simulink model "BaseEngineController_LS"  (Simulink 7.7)
settings: Solver=FixedStepDiscrete  StartTime=0.0  StopTime=10.0  RelTol=1e-3
PreLoadFcn:
  | try, eval([bdroot '_setup']); catch, eval('model_setup', ''); end
InitFcn:
  | try, eval([bdroot '_setup']); catch, eval('model_setup', ''); end
undefined symbols (not defined in the file): ECU555, High, motohawk_build_version, motohawk_trunc_name, motohawk_vardec_config_group, motohawk_vardec_path, True
libraries: MotoHawk_lib x1418, motohawk_control_primitives_lib x183, motohawk_engine_lib x32, simulink x21, motohawk_annotations_lib x9, AutoDoc_lib x8, simulink_extras x4, motohawk_ccp_examples_lib x1, motohawk_control_primitives_motoshare_lib x1
(part 14 of 27)

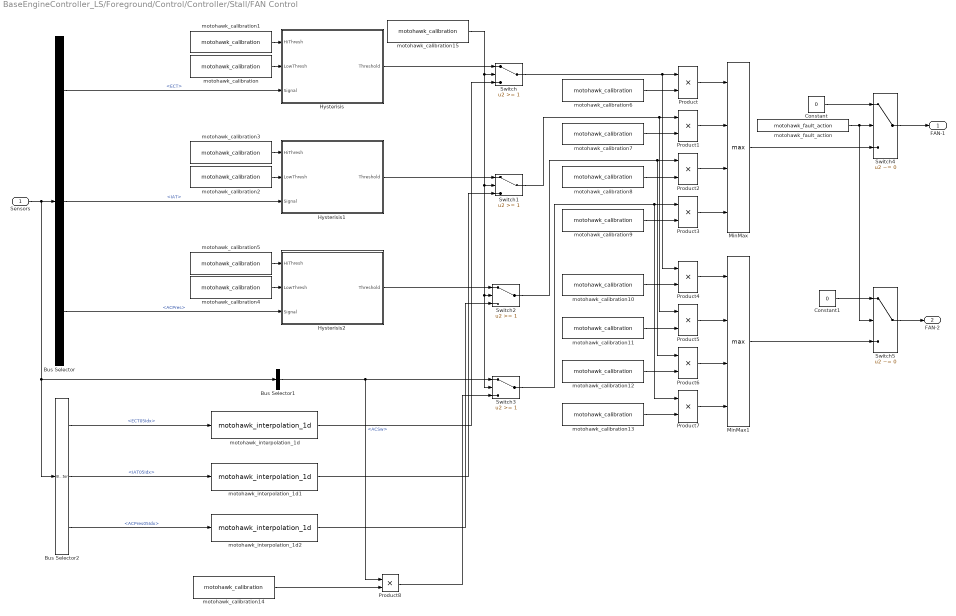
== system BaseEngineController_LS/Foreground/Control/Controller/Stall/FAN Control ==
  Sensors : Inport
  Bus Selector : BusSelector  OutputSignals=Raw.NonLinearSensors.ECT,Raw.NonLinearSensors.IAT,Raw.LinearSensors.ACPres
  Bus Selector1 : BusSelector  OutputSignals=Raw.Digital.ACSw
  Bus Selector2 : BusSelector  OutputSignals=RawIndexes.ECT05Idx,RawIndexes.IAT05Idx,RawIndexes.ACPres05Idx
  Constant : Constant  Value=0
  Constant1 : Constant  Value=0
  Hysterisis : Subsystem  AncestorBlock=motohawk_control_primitives_lib/Hysterisis
      mask Display:
      | patch([0 0 1 1], [0 0.075 0.075 0], [230/255 0/255 0/255])
      | patch([0 0 1 1], [0.025 0.05 0.05 0.025], [150/255 0/255 0/255])
      | patch([0 0 1 1], [0 0.025 0.025 0], [0/255 0/255 0/255])
      | 
      | disp('HYSTERISIS')
  Hysterisis1 : Subsystem  AncestorBlock=motohawk_control_primitives_lib/Hysterisis
      mask Display:
      | patch([0 0 1 1], [0 0.075 0.075 0], [230/255 0/255 0/255])
      | patch([0 0 1 1], [0.025 0.05 0.05 0.025], [150/255 0/255 0/255])
      | patch([0 0 1 1], [0 0.025 0.025 0], [0/255 0/255 0/255])
      | 
      | disp('HYSTERISIS')
  Hysterisis2 : Subsystem  AncestorBlock=motohawk_control_primitives_lib/Hysterisis
      mask Display:
      | patch([0 0 1 1], [0 0.075 0.075 0], [230/255 0/255 0/255])
      | patch([0 0 1 1], [0.025 0.05 0.05 0.025], [150/255 0/255 0/255])
      | patch([0 0 1 1], [0 0.025 0.025 0], [0/255 0/255 0/255])
      | 
      | disp('HYSTERISIS')
  MinMax : MinMax  Function=max  Inputs=4
  MinMax1 : MinMax  Function=max  Inputs=4
  Product{,1..8} (9 alike) : Product  RndMeth=Zero
  Switch{,1..3} (4 alike) : Switch  Threshold=1
  Switch4 : Switch  Criteria=u2 ~= 0
  Switch5 : Switch  Criteria=u2 ~= 0
  motohawk_calibration : MotoHawk_lib/Calibration & Probing Blocks/motohawk_calibration  nam='ECTFanOff'  val=80  storage=Calibration  show_more=on  name_source=Use Parameter  data_type=Inherit from 'Default Value'  read_level=1  write_level=1  ovr_cals=on  view_as=Number  enum_struct={'Disabled', 'Enabled'}  vector_style=Wide Row  use_help_units=on  help='ECT temp when the fan turns off'  units='degC'  use_header_enum=off  row_header_enum={}  col_header_enum={}  use_min_max=off  min_val=-inf  max_val=inf  use_precision=off  precision=''  gain=1  offset=0  exp=1  use_mototune_group=off  mototune_group=motohawk_vardec_path(gcb)
  motohawk_calibration1 : MotoHawk_lib/Calibration & Probing Blocks/motohawk_calibration  nam='ECTFanOn'  val=90  storage=Calibration  show_more=on  name_source=Use Parameter  data_type=Inherit from 'Default Value'  read_level=1  write_level=1  ovr_cals=on  view_as=Number  enum_struct={'Disabled', 'Enabled'}  vector_style=Wide Row  use_help_units=on  help='ECT temp when the fan turns on'  units='degC'  use_header_enum=off  row_header_enum={}  col_header_enum={}  use_min_max=off  min_val=-inf  max_val=inf  use_precision=off  precision=''  gain=1  offset=0  exp=1  use_mototune_group=off  mototune_group=motohawk_vardec_path(gcb)
  motohawk_calibration10 : MotoHawk_lib/Calibration & Probing Blocks/motohawk_calibration  nam='Fan2ECT'  val=1  storage=Calibration  show_more=on  name_source=Use Parameter  data_type=boolean  read_level=1  write_level=1  ovr_cals=on  view_as=Enumeration  enum_struct={'Disabled', 'Enabled'}  vector_style=Wide Row  use_help_units=on  help='Fan Enabler'  units=''  use_header_enum=off  row_header_enum={}  col_header_enum={}  use_min_max=off  min_val=-inf  max_val=inf  use_precision=off  precision=''  gain=1  offset=0  exp=1  use_mototune_group=off  mototune_group=motohawk_vardec_path(gcb)
  motohawk_calibration11 : MotoHawk_lib/Calibration & Probing Blocks/motohawk_calibration  nam='Fan2IAT'  val=0  storage=Calibration  show_more=on  name_source=Use Parameter  data_type=boolean  read_level=1  write_level=1  ovr_cals=on  view_as=Enumeration  enum_struct={'Disabled', 'Enabled'}  vector_style=Wide Row  use_help_units=on  help='Fan Enabler'  units=''  use_header_enum=off  row_header_enum={}  col_header_enum={}  use_min_max=off  min_val=-inf  max_val=inf  use_precision=off  precision=''  gain=1  offset=0  exp=1  use_mototune_group=off  mototune_group=motohawk_vardec_path(gcb)
  motohawk_calibration12 : MotoHawk_lib/Calibration & Probing Blocks/motohawk_calibration  nam='Fan2ACPres'  val=0  storage=Calibration  show_more=on  name_source=Use Parameter  data_type=boolean  read_level=1  write_level=1  ovr_cals=on  view_as=Enumeration  enum_struct={'Disabled', 'Enabled'}  vector_style=Wide Row  use_help_units=on  help='Fan Enabler'  units=''  use_header_enum=off  row_header_enum={}  col_header_enum={}  use_min_max=off  min_val=-inf  max_val=inf  use_precision=off  precision=''  gain=1  offset=0  exp=1  use_mototune_group=off  mototune_group=motohawk_vardec_path(gcb)
  motohawk_calibration13 : MotoHawk_lib/Calibration & Probing Blocks/motohawk_calibration  nam='Fan2ACSw'  val=0  storage=Calibration  show_more=on  name_source=Use Parameter  data_type=boolean  read_level=1  write_level=1  ovr_cals=on  view_as=Enumeration  enum_struct={'Disabled', 'Enabled'}  vector_style=Wide Row  use_help_units=on  help='Fan Enabler'  units=''  use_header_enum=off  row_header_enum={}  col_header_enum={}  use_min_max=off  min_val=-inf  max_val=inf  use_precision=off  precision=''  gain=1  offset=0  exp=1  use_mototune_group=off  mototune_group=motohawk_vardec_path(gcb)
  motohawk_calibration14 : MotoHawk_lib/Calibration & Probing Blocks/motohawk_calibration  nam='ACSwFanSpeed_Stall'  val=50  storage=Calibration  show_more=on  name_source=Use Parameter  data_type=double  read_level=1  write_level=1  ovr_cals=on  view_as=Number  enum_struct={'Disabled', 'Enabled'}  vector_style=Wide Row  use_help_units=on  help='Fan speed % req for AC Sw 0 to disable'  units='%'  use_header_enum=off  row_header_enum={}  col_header_enum={}  use_min_max=on  min_val=0  max_val=100  use_precision=off  precision=''  gain=1  offset=0  exp=1  use_mototune_group=off  mototune_group=motohawk_vardec_path(gcb)
  motohawk_calibration15 : MotoHawk_lib/Calibration & Probing Blocks/motohawk_calibration  nam='FAN_Mode'  val=0  storage=Calibration  show_more=on  name_source=Use Parameter  data_type=boolean  read_level=1  write_level=1  ovr_cals=on  view_as=Enumeration  enum_struct={'PWM', 'OnOff'}  vector_style=Wide Row  use_help_units=on  help=''  units=''  use_header_enum=off  row_header_enum={}  col_header_enum={}  use_min_max=off  min_val=-inf  max_val=inf  use_precision=off  precision=''  gain=1  offset=0  exp=1  use_mototune_group=off  mototune_group=motohawk_vardec_path(gcb)
  motohawk_calibration2 : MotoHawk_lib/Calibration & Probing Blocks/motohawk_calibration  nam='IATFanOff'  val=80  storage=Calibration  show_more=on  name_source=Use Parameter  data_type=Inherit from 'Default Value'  read_level=1  write_level=1  ovr_cals=on  view_as=Number  enum_struct={'Disabled', 'Enabled'}  vector_style=Wide Row  use_help_units=on  help='IAT temp when the fan turns off'  units='degC'  use_header_enum=off  row_header_enum={}  col_header_enum={}  use_min_max=off  min_val=-inf  max_val=inf  use_precision=off  precision=''  gain=1  offset=0  exp=1  use_mototune_group=off  mototune_group=motohawk_vardec_path(gcb)
  motohawk_calibration3 : MotoHawk_lib/Calibration & Probing Blocks/motohawk_calibration  nam='IATFanOn'  val=90  storage=Calibration  show_more=on  name_source=Use Parameter  data_type=Inherit from 'Default Value'  read_level=1  write_level=1  ovr_cals=on  view_as=Number  enum_struct={'Disabled', 'Enabled'}  vector_style=Wide Row  use_help_units=on  help='IAT temp when the fan turns on'  units='degC'  use_header_enum=off  row_header_enum={}  col_header_enum={}  use_min_max=off  min_val=-inf  max_val=inf  use_precision=off  precision=''  gain=1  offset=0  exp=1  use_mototune_group=off  mototune_group=motohawk_vardec_path(gcb)
  motohawk_calibration4 : MotoHawk_lib/Calibration & Probing Blocks/motohawk_calibration  nam='ACPresFanOff'  val=2000  storage=Calibration  show_more=on  name_source=Use Parameter  data_type=Inherit from 'Default Value'  read_level=1  write_level=1  ovr_cals=on  view_as=Number  enum_struct={'Disabled', 'Enabled'}  vector_style=Wide Row  use_help_units=on  help='AC pressure when the fan turns off'  units='kpa'  use_header_enum=off  row_header_enum={}  col_header_enum={}  use_min_max=off  min_val=-inf  max_val=inf  use_precision=off  precision=''  gain=1  offset=0  exp=1  use_mototune_group=off  mototune_group=motohawk_vardec_path(gcb)
  motohawk_calibration5 : MotoHawk_lib/Calibration & Probing Blocks/motohawk_calibration  nam='ACPresFanOn'  val=2500  storage=Calibration  show_more=on  name_source=Use Parameter  data_type=Inherit from 'Default Value'  read_level=1  write_level=1  ovr_cals=on  view_as=Number  enum_struct={'Disabled', 'Enabled'}  vector_style=Wide Row  use_help_units=on  help='AC pressure when the fan turns on'  units='kpa'  use_header_enum=off  row_header_enum={}  col_header_enum={}  use_min_max=off  min_val=-inf  max_val=inf  use_precision=off  precision=''  gain=1  offset=0  exp=1  use_mototune_group=off  mototune_group=motohawk_vardec_path(gcb)
  motohawk_calibration6 : MotoHawk_lib/Calibration & Probing Blocks/motohawk_calibration  nam='Fan1ECT'  val=1  storage=Calibration  show_more=on  name_source=Use Parameter  data_type=boolean  read_level=1  write_level=1  ovr_cals=on  view_as=Enumeration  enum_struct={'Disabled', 'Enabled'}  vector_style=Wide Row  use_help_units=on  help='Fan Enabler'  units=''  use_header_enum=off  row_header_enum={}  col_header_enum={}  use_min_max=off  min_val=-inf  max_val=inf  use_precision=off  precision=''  gain=1  offset=0  exp=1  use_mototune_group=off  mototune_group=motohawk_vardec_path(gcb)
  motohawk_calibration7 : MotoHawk_lib/Calibration & Probing Blocks/motohawk_calibration  nam='Fan1IAT'  val=0  storage=Calibration  show_more=on  name_source=Use Parameter  data_type=boolean  read_level=1  write_level=1  ovr_cals=on  view_as=Enumeration  enum_struct={'Disabled', 'Enabled'}  vector_style=Wide Row  use_help_units=on  help='Fan Enabler'  units=''  use_header_enum=off  row_header_enum={}  col_header_enum={}  use_min_max=off  min_val=-inf  max_val=inf  use_precision=off  precision=''  gain=1  offset=0  exp=1  use_mototune_group=off  mototune_group=motohawk_vardec_path(gcb)
  motohawk_calibration8 : MotoHawk_lib/Calibration & Probing Blocks/motohawk_calibration  nam='Fan1ACPres'  val=0  storage=Calibration  show_more=on  name_source=Use Parameter  data_type=boolean  read_level=1  write_level=1  ovr_cals=on  view_as=Enumeration  enum_struct={'Disabled', 'Enabled'}  vector_style=Wide Row  use_help_units=on  help='Fan Enabler'  units=''  use_header_enum=off  row_header_enum={}  col_header_enum={}  use_min_max=off  min_val=-inf  max_val=inf  use_precision=off  precision=''  gain=1  offset=0  exp=1  use_mototune_group=off  mototune_group=motohawk_vardec_path(gcb)
  motohawk_calibration9 : MotoHawk_lib/Calibration & Probing Blocks/motohawk_calibration  nam='Fan1ACSw'  val=0  storage=Calibration  show_more=on  name_source=Use Parameter  data_type=boolean  read_level=1  write_level=1  ovr_cals=on  view_as=Enumeration  enum_struct={'Disabled', 'Enabled'}  vector_style=Wide Row  use_help_units=on  help='Fan Enabler'  units=''  use_header_enum=off  row_header_enum={}  col_header_enum={}  use_min_max=off  min_val=-inf  max_val=inf  use_precision=off  precision=''  gain=1  offset=0  exp=1  use_mototune_group=off  mototune_group=motohawk_vardec_path(gcb)
  motohawk_fault_action : MotoHawk_lib/Fault Management Blocks/motohawk_fault_action  nam='DisableFanStall'  output_status=on  eval_nam=DisableFanStall
  motohawk_interpolation_1d : MotoHawk_lib/Lookup Tables/motohawk_interpolation_1d  nam='ECTFanSpeed_Stall'  table_data=[1 2 3 4 5]  show_more=off  data_type=Inherit from 'Table Data'  storage=NonAdaptive  read_level=1  write_level=1  ovr_cals=on  use_help=off  help=''  units=''  use_min_max=off  min_val=-inf  max_val=inf  use_precision=off  precision=''  gain=1  offset=0  exp=1  use_links=off  prelookup_block=''  output_name=''  use_mototune_group=off  mototune_group=motohawk_vardec_path(gcb)
  motohawk_interpolation_1d1 : MotoHawk_lib/Lookup Tables/motohawk_interpolation_1d  nam='IATFanSpeed_Stall'  table_data=[1 2 3 4 5]  show_more=off  data_type=Inherit from 'Table Data'  storage=NonAdaptive  read_level=1  write_level=1  ovr_cals=on  use_help=off  help=''  units=''  use_min_max=off  min_val=-inf  max_val=inf  use_precision=off  precision=''  gain=1  offset=0  exp=1  use_links=off  prelookup_block=''  output_name=''  use_mototune_group=off  mototune_group=motohawk_vardec_path(gcb)
  motohawk_interpolation_1d2 : MotoHawk_lib/Lookup Tables/motohawk_interpolation_1d  nam='ACPresFanSpeed_Stall'  table_data=[1 2 3 4 5]  show_more=off  data_type=Inherit from 'Table Data'  storage=NonAdaptive  read_level=1  write_level=1  ovr_cals=on  use_help=off  help=''  units=''  use_min_max=off  min_val=-inf  max_val=inf  use_precision=off  precision=''  gain=1  offset=0  exp=1  use_links=off  prelookup_block=''  output_name=''  use_mototune_group=off  mototune_group=motohawk_vardec_path(gcb)
  FAN-1 : Outport
  FAN-2 : Outport  Port=2
  wires:
  Sensors/1 -> Bus Selector/1, Bus Selector1/1, Bus Selector2/1
  Bus Selector/1 -> Hysterisis/3(Signal)  "<ECT>"
  motohawk_calibration/1 -> Hysterisis/2(LowThresh)
  motohawk_calibration1/1 -> Hysterisis/1(HiThresh)
  motohawk_calibration3/1 -> Hysterisis1/1(HiThresh)
  Bus Selector/2 -> Hysterisis1/3(Signal)  "<IAT>"
  motohawk_calibration2/1 -> Hysterisis1/2(LowThresh)
  Bus Selector/3 -> Hysterisis2/3(Signal)  "<ACPres>"
  motohawk_calibration4/1 -> Hysterisis2/2(LowThresh)
  motohawk_calibration5/1 -> Hysterisis2/1(HiThresh)
  Product/1 -> MinMax/1
  motohawk_calibration6/1 -> Product/2
  Product1/1 -> MinMax/2
  motohawk_calibration7/1 -> Product1/2
  Product2/1 -> MinMax/3
  motohawk_calibration8/1 -> Product2/2
  Product3/1 -> MinMax/4
  motohawk_calibration9/1 -> Product3/2
  Bus Selector1/1 -> Product8/1, Switch3/1  "<ACSw>"
  Product4/1 -> MinMax1/1
  motohawk_calibration10/1 -> Product4/2
  Product5/1 -> MinMax1/2
  motohawk_calibration11/1 -> Product5/2
  Product6/1 -> MinMax1/3
  motohawk_calibration12/1 -> Product6/2
  Product7/1 -> MinMax1/4
  motohawk_calibration13/1 -> Product7/2
  motohawk_calibration14/1 -> Product8/2
  Hysterisis/1(Threshold) -> Switch/1
  motohawk_calibration15/1 -> Switch/2, Switch1/2, Switch2/2, Switch3/2
  Hysterisis1/1(Threshold) -> Switch1/1
  Hysterisis2/1(Threshold) -> Switch2/1
  motohawk_interpolation_1d/1 -> Switch/3
  motohawk_interpolation_1d1/1 -> Switch1/3
  motohawk_interpolation_1d2/1 -> Switch2/3
  Product8/1 -> Switch3/3
  Switch/1 -> Product/1, Product4/1
  Switch1/1 -> Product1/1, Product5/1
  Switch2/1 -> Product2/1, Product6/1
  Switch3/1 -> Product3/1, Product7/1
  MinMax/1 -> Switch4/3
  motohawk_fault_action/1 -> Switch4/2, Switch5/2
  Constant/1 -> Switch4/1
  MinMax1/1 -> Switch5/3
  Constant1/1 -> Switch5/1
  Switch4/1 -> FAN-1/1
  Switch5/1 -> FAN-2/1
  Bus Selector2/1 -> motohawk_interpolation_1d/1  "<ECT05Idx>"
  Bus Selector2/2 -> motohawk_interpolation_1d1/1  "<IAT05Idx>"
  Bus Selector2/3 -> motohawk_interpolation_1d2/1  "<ACPres05Idx>"

== system BaseEngineController_LS/Foreground/Control/Controller/Stall/Fuel Pump at Startup ==
  note: Turn On Fuel Pump
      | for 'StartupTime' seconds
  note: Turn on Fuel Pump at Startup
  Constant : Constant  OutDataTypeStr=boolean
  Relational Operator : RelationalOperator  Operator=<  ZeroCross=off  InputSameDT=on
  Switch : Switch  Criteria=u2 > Threshold
  Time Since Enabled : motohawk_control_primitives_lib/Time Since Enabled  SystemSampleTime=-1  samp_time=.005
  motohawk_calibration : MotoHawk_lib/Calibration & Probing Blocks/motohawk_calibration  nam='FuelPumpStartTime'  val=3  storage=Calibration  show_more=on  name_source=Use Parameter  data_type=Inherit from 'Default Value'  read_level=1  write_level=1  ovr_cals=on  view_as=Number  enum_struct={'Disabled', 'Enabled'}  vector_style=Wide Row  use_help_units=on  help='The length of time for the Fuel Pump relay to be enabled at startup'  units='sec'  use_header_enum=off  row_header_enum={}  col_header_enum={}  use_min_max=on  min_val=0  max_val=100  use_precision=off  precision=''  gain=1  offset=0  exp=1  use_mototune_group=on  mototune_group=motohawk_vardec_path(gcb)
  motohawk_calibration1 : MotoHawk_lib/Calibration & Probing Blocks/motohawk_calibration  nam='Constant_Fuel_Pump'  val=0  storage=Calibration  show_more=on  name_source=Use Parameter  data_type=boolean  read_level=1  write_level=1  ovr_cals=on  view_as=Number  enum_struct={'Disabled', 'Enabled'}  vector_style=Wide Row  use_help_units=off  help=''  units=''  use_header_enum=off  row_header_enum={}  col_header_enum={}  use_min_max=off  min_val=-inf  max_val=inf  use_precision=off  precision=''  gain=1  offset=0  exp=1  use_mototune_group=off  mototune_group=motohawk_vardec_path(gcb)
  motohawk_probe : MotoHawk_lib/Calibration & Probing Blocks/motohawk_probe  nam='FuelPumpTSE'  show_more=on  name_source=Use Parameter  read_level=1  view_as=Number  enum_struct={'Disabled', 'Enabled'}  vector_style=Wide Row  use_help_units=on  help=''  units=''  use_header_enum=off  row_header_enum={}  col_header_enum={}  use_precision=on  precision=''  gain=1  offset=0  exp=1  use_mototune_group=on  mototune_group=motohawk_vardec_path(gcb)
  FUELP [bool] : Outport
  wires:
  Time Since Enabled/1 -> Relational Operator/1, motohawk_probe/1
  motohawk_calibration/1 -> Relational Operator/2
  motohawk_calibration1/1 -> Switch/2
  Switch/1 -> FUELP [bool]/1
  Relational Operator/1 -> Switch/3
  Constant/1 -> Switch/1

== system BaseEngineController_LS/Foreground/Control/Controller/Stall/Stall Throttle ==
  Sensors : Inport
  Bus Selector : BusSelector  OutputSignals=RawProcessed.TimeSinceKeyOn
  Bus Selector1 : BusSelector  OutputSignals=RawProcessed.APPPcnt
  Ice Break : Stateflow chart  TreatAsAtomicUnit=on
  Product1 : Product  Inputs=3  RndMeth=Zero
  Product2 : Product  RndMeth=Zero
  Relational Operator2 : RelationalOperator  OutDataTypeStr=boolean
  Relational Operator3 : RelationalOperator  OutDataTypeStr=boolean
  Switch : Switch  Criteria=u2 ~= 0
  Time Since Enabled (With Input)2 : motohawk_control_primitives_lib/Time Since Enabled (With Input)1  SystemSampleTime=-1  nam='AppStallOvrTmr'  samp_time=-1  init=0  upperlim=16000
  motohawk_calibration : MotoHawk_lib/Calibration & Probing Blocks/motohawk_calibration  nam='ETC_IceBreakPos'  val=100  storage=Calibration  show_more=on  name_source=Use Parameter  data_type=Inherit from 'Default Value'  read_level=1  write_level=1  ovr_cals=on  view_as=Number  enum_struct={'Disabled', 'Enabled'}  vector_style=Wide Row  use_help_units=on  help=''  units='%'  use_header_enum=off  row_header_enum={}  col_header_enum={}  use_min_max=on  min_val=0  max_val=100  use_precision=off  precision=''  gain=1  offset=0  exp=1  use_mototune_group=off  mototune_group=motohawk_vardec_path(gcb)
  motohawk_calibration1 : MotoHawk_lib/Calibration & Probing Blocks/motohawk_calibration  nam='ETC_IceBreakEnblTm'  val=1  storage=Calibration  show_more=on  name_source=Use Parameter  data_type=Inherit from 'Default Value'  read_level=1  write_level=1  ovr_cals=on  view_as=Number  enum_struct={'Disabled', 'Enabled'}  vector_style=Wide Row  use_help_units=on  help=''  units='sec'  use_header_enum=off  row_header_enum={}  col_header_enum={}  use_min_max=on  min_val=0  max_val=10  use_precision=off  precision=''  gain=1  offset=0  exp=1  use_mototune_group=off  mototune_group=motohawk_vardec_path(gcb)
  motohawk_calibration2 : MotoHawk_lib/Calibration & Probing Blocks/motohawk_calibration  nam='ETC_IceBreakHoldTm'  val=.2  storage=Calibration  show_more=on  name_source=Use Parameter  data_type=Inherit from 'Default Value'  read_level=1  write_level=1  ovr_cals=on  view_as=Number  enum_struct={'Disabled', 'Enabled'}  vector_style=Wide Row  use_help_units=on  help=''  units='sec'  use_header_enum=off  row_header_enum={}  col_header_enum={}  use_min_max=on  min_val=0  max_val=10  use_precision=off  precision=''  gain=1  offset=0  exp=1  use_mototune_group=off  mototune_group=motohawk_vardec_path(gcb)
  motohawk_calibration3 : MotoHawk_lib/Calibration & Probing Blocks/motohawk_calibration  nam='ETC_StallAppOvrThesh'  val=20  storage=Calibration  show_more=on  name_source=Use Parameter  data_type=Inherit from 'Default Value'  read_level=1  write_level=1  ovr_cals=on  view_as=Number  enum_struct={'Disabled', 'Enabled'}  vector_style=Wide Row  use_help_units=on  help=''  units='%'  use_header_enum=off  row_header_enum={}  col_header_enum={}  use_min_max=on  min_val=0  max_val=100  use_precision=off  precision=''  gain=1  offset=0  exp=1  use_mototune_group=off  mototune_group=motohawk_vardec_path(gcb)
  motohawk_calibration4 : MotoHawk_lib/Calibration & Probing Blocks/motohawk_calibration  nam='ETC_StallAppOvrTm'  val=.2  storage=Calibration  show_more=on  name_source=Use Parameter  data_type=Inherit from 'Default Value'  read_level=1  write_level=1  ovr_cals=on  view_as=Number  enum_struct={'Disabled', 'Enabled'}  vector_style=Wide Row  use_help_units=on  help=''  units='sec'  use_header_enum=off  row_header_enum={}  col_header_enum={}  use_min_max=on  min_val=0  max_val=10  use_precision=off  precision=''  gain=1  offset=0  exp=1  use_mototune_group=off  mototune_group=motohawk_vardec_path(gcb)
  motohawk_probe : MotoHawk_lib/Calibration & Probing Blocks/motohawk_probe  nam='ETCStallReq'  show_more=on  name_source=Use Parameter  read_level=1  view_as=Number  enum_struct={'Disabled', 'Enabled'}  vector_style=Wide Row  use_help_units=on  help=''  units='%'  use_header_enum=off  row_header_enum={}  col_header_enum={}  use_precision=off  precision=''  gain=1  offset=0  exp=1  use_mototune_group=off  mototune_group=motohawk_vardec_path(gcb)
  motohawk_probe1 : MotoHawk_lib/Calibration & Probing Blocks/motohawk_probe  nam='ETCStallAppOvrReq'  show_more=on  name_source=Use Parameter  read_level=1  view_as=Number  enum_struct={'Disabled', 'Enabled'}  vector_style=Wide Row  use_help_units=on  help=''  units='%'  use_header_enum=off  row_header_enum={}  col_header_enum={}  use_precision=off  precision=''  gain=1  offset=0  exp=1  use_mototune_group=off  mototune_group=motohawk_vardec_path(gcb)
  motohawk_probe2 : MotoHawk_lib/Calibration & Probing Blocks/motohawk_probe  nam='ETCStallIceBreakReq'  show_more=on  name_source=Use Parameter  read_level=1  view_as=Number  enum_struct={'Disabled', 'Enabled'}  vector_style=Wide Row  use_help_units=on  help=''  units='%'  use_header_enum=off  row_header_enum={}  col_header_enum={}  use_precision=off  precision=''  gain=1  offset=0  exp=1  use_mototune_group=off  mototune_group=motohawk_vardec_path(gcb)
  ETC % : Outport
  wires:
  Sensors/1 -> Bus Selector/1, Bus Selector1/1
  Bus Selector1/1 -> Relational Operator2/1, Product1/3  "<APPPcnt>"
  motohawk_calibration3/1 -> Relational Operator2/2
  Relational Operator2/1 -> Time Since Enabled (With Input)2/1, Product1/2, Product2/2
  Time Since Enabled (With Input)2/1 -> Relational Operator3/1
  motohawk_calibration4/1 -> Relational Operator3/2
  Relational Operator3/1 -> Product1/1, Product2/1
  Product2/1 -> Switch/2
  Product1/1 -> Switch/1, motohawk_probe1/1
  Ice Break/1(etc) -> Switch/3, motohawk_probe2/1
  Switch/1 -> ETC %/1, motohawk_probe/1
  Bus Selector/1 -> Ice Break/1(timeSinceKeyOn)  "<TimeSinceKeyOn>"
  motohawk_calibration1/1 -> Ice Break/2(enblTime)
  motohawk_calibration2/1 -> Ice Break/3(hldTime)
  motohawk_calibration/1 -> Ice Break/4(icePos)

== system BaseEngineController_LS/Foreground/Control/Diagnostics/Fuel Economy/Calculate Fuel Density ==
  Ethanol_xx [%] : Inport
  " " : Constant  Value=1.0
  " Ethanol density (g/ml)" : Constant  Value=.789
  " Gasoline density (g/ml)" : Constant  Value=0.737
  Add : Sum
  Add1 : Sum  Inputs=+-
  Gain : Gain  Gain=.01
  Product1 : Product  RndMeth=Zero
  Product2 : Product  RndMeth=Zero
  Fuel Density (g/ml) : Outport
  wires:
  " Ethanol density (g/ml)"/1 -> Product2/1
  " Gasoline density (g/ml)"/1 -> Product1/1
  Product1/1 -> Add/1
  Product2/1 -> Add/2
  Add/1 -> Fuel Density (g/ml)/1
  Gain/1 -> Product2/2, Add1/2
  Add1/1 -> Product1/2
  " "/1 -> Add1/1
  Ethanol_xx [%]/1 -> Gain/1

== system BaseEngineController_LS/Foreground/Control/Diagnostics/Fuel Economy/First Order Low Pass (Tunable) ==
  note: Tunable 1st-Order Low-Pass Filter
  in : Inport
  First Order Low Pass : motohawk_control_primitives_lib/First Order Low Pass  SystemSampleTime=-1
  MinMax : MinMax  Function=max  Inputs=2  SaturateOnIntegerOverflow=on  InputSameDT=on
  Product : Product  Inputs=*/  SaturateOnIntegerOverflow=on  InputSameDT=on  OutDataTypeStr=Inherit: Same as first input
  motohawk_calibration2 : MotoHawk_lib/Calibration & Probing Blocks/motohawk_calibration  nam='FuelEconomy_FilterC'  val=1  storage=Calibration  show_more=on  name_source=Use Parameter  data_type=Inherit from 'Default Value'  read_level=1  write_level=1  ovr_cals=on  view_as=Number  enum_struct={'Disabled', 'Enabled'}  vector_style=Wide Row  use_help_units=on  help='Time constant for fuel economy filter'  units='Time const'  use_header_enum=off  row_header_enum={}  col_header_enum={}  use_min_max=on  min_val=0.001  max_val=100  use_precision=off  precision=''  gain=1  offset=0  exp=1  use_mototune_group=on  mototune_group=motohawk_vardec_path(gcb)
  motohawk_delta_time : MotoHawk_lib/Extra Development Blocks/motohawk_delta_time  samp_time=samp_time  init_val=0  mode=Seconds (double)
  out : Outport
  wires:
  First Order Low Pass/1 -> out/1
  in/1 -> First Order Low Pass/1
  motohawk_delta_time/1 -> Product/1, MinMax/1
  Product/1 -> First Order Low Pass/2
  MinMax/1 -> Product/2
  motohawk_calibration2/1 -> MinMax/2

== system BaseEngineController_LS/Foreground/Control/Diagnostics/MISFIRE/MisfireDiagSub ==
  Enable : EnablePort
  MisfireDiagFunc : Subsystem  TreatAsAtomicUnit=on
  motohawk_trigger : MotoHawk_lib/Trigger Blocks/motohawk_trigger  Tag=Trigger  trigger=FGND_HIRES  function_name=Trigger_FGND_HIRES_33246p001  priority_order=1  inherited=on  run_disabled=off  override_app_monitor=off  target=ECU555_80
  wires:
  motohawk_trigger/1 -> MisfireDiagFunc/Trigger

== system BaseEngineController_LS/Foreground/Control/Diagnostics/O2 Smart Sensor/Bank2Bank ==
  Sensors : Inport
  DesEquivRatio : Inport  Port=2
  Abs : Abs
  Bus Selector : BusSelector  OutputSignals=RawProcessed.TimeSinceRun
  Bus Selector1 : BusSelector  OutputSignals=Raw.NonLinearSensors.ECT
  Bus Selector2 : BusSelector  OutputSignals=Raw.CAN.O2_BUS.BANK1.DataValidState,Raw.CAN.O2_BUS.BANK2.DataValidState
  Bus Selector3 : BusSelector  OutputSignals=DesEquivRatio
  Bus Selector4 : BusSelector  OutputSignals=DesEquivRatio
  Bus Selector5 : BusSelector  OutputSignals=RawIndexes.RPM09Idx,RawIndexes.MAP09Idx
  Bus Selector6 : BusSelector  OutputSignals=Raw.CAN.O2_BankA,Raw.CAN.O2_BankB
  Logical Operator : Logic  Inputs=8  AllPortsSameDT=off  OutDataTypeStr=boolean
  Logical Operator1 : Logic  AllPortsSameDT=off  OutDataTypeStr=boolean
  Logical Operator10 : Logic  Operator=NOT  Inputs=3  AllPortsSameDT=off  OutDataTypeStr=boolean
  Logical Operator33 : Logic  Operator=NOT  Inputs=3  AllPortsSameDT=off  OutDataTypeStr=boolean
  Logical Operator34 : Logic  Operator=OR  Inputs=5  AllPortsSameDT=off  OutDataTypeStr=boolean
  Relational Operator{,1..2,4} (4 alike) : RelationalOperator  OutDataTypeStr=boolean
  Relational Operator3 : RelationalOperator  Operator=<=  OutDataTypeStr=boolean
  Run State : motohawk_control_primitives_lib/CompareTo  SystemSampleTime=-1  op===  val=3
  Sum : Sum  Inputs=+-
  motohawk_calibration : MotoHawk_lib/Calibration & Probing Blocks/motohawk_calibration  nam='O2Diag_Bank2Bank_MinRunTime'  val=30  storage=Calibration  show_more=off  name_source=Use Parameter  data_type=Inherit from 'Default Value'  read_level=1  write_level=1  ovr_cals=on  view_as=Number  enum_struct={'Disabled', 'Enabled'}  vector_style=Wide Row  use_help_units=off  help=''  units=''  use_header_enum=off  row_header_enum={}  col_header_enum={}  use_min_max=off  min_val=-inf  max_val=inf  use_precision=off  precision=''  gain=1  offset=0  exp=1  use_mototune_group=off  mototune_group=motohawk_vardec_path(gcb)
  motohawk_calibration1 : MotoHawk_lib/Calibration & Probing Blocks/motohawk_calibration  nam='O2Diag_Bank2Bank_MinECT'  val=60  storage=Calibration  show_more=on  name_source=Use Parameter  data_type=int16  read_level=1  write_level=1  ovr_cals=on  view_as=Number  enum_struct={'Disabled', 'Enabled'}  vector_style=Wide Row  use_help_units=off  help=''  units=''  use_header_enum=off  row_header_enum={}  col_header_enum={}  use_min_max=off  min_val=-inf  max_val=inf  use_precision=off  precision=''  gain=1  offset=0  exp=1  use_mototune_group=off  mototune_group=motohawk_vardec_path(gcb)
  motohawk_calibration2 : MotoHawk_lib/Calibration & Probing Blocks/motohawk_calibration  nam='O2Diag_Bank2Bank_MinDesEquivRatio'  val=.5  storage=Calibration  show_more=on  name_source=Use Parameter  data_type=double  read_level=1  write_level=1  ovr_cals=on  view_as=Number  enum_struct={'Disabled', 'Enabled'}  vector_style=Wide Row  use_help_units=off  help=''  units=''  use_header_enum=off  row_header_enum={}  col_header_enum={}  use_min_max=off  min_val=-inf  max_val=inf  use_precision=off  precision=''  gain=1  offset=0  exp=1  use_mototune_group=off  mototune_group=motohawk_vardec_path(gcb)
  motohawk_calibration3 : MotoHawk_lib/Calibration & Probing Blocks/motohawk_calibration  nam='O2Diag_Bank2Bank_MaxDesEquivRatio'  val=1.5  storage=Calibration  show_more=on  name_source=Use Parameter  data_type=double  read_level=1  write_level=1  ovr_cals=on  view_as=Number  enum_struct={'Disabled', 'Enabled'}  vector_style=Wide Row  use_help_units=off  help=''  units=''  use_header_enum=off  row_header_enum={}  col_header_enum={}  use_min_max=off  min_val=-inf  max_val=inf  use_precision=off  precision=''  gain=1  offset=0  exp=1  use_mototune_group=off  mototune_group=motohawk_vardec_path(gcb)
  motohawk_data_read : MotoHawk_lib/Data Storage Blocks/motohawk_data_read  source=Lookup By Name  structure=Scalar  operation=Read scalar from location by index  sz_vec=4  sz_row=2  sz_col=3  typ=boolean  nam='BankB_Enbl'  checkNull=on  struct_inst_name='MyData'  struct_nam='MyStruct'
  motohawk_data_read1 : MotoHawk_lib/Data Storage Blocks/motohawk_data_read  source=Lookup By Name  structure=Scalar  operation=Read entire data structure at once  sz_vec=4  sz_row=2  sz_col=3  typ=uint8  nam='EngineState'  checkNull=on  struct_inst_name='Struct1'  struct_nam='MyStruct'
  motohawk_fault_def6 : MotoHawk_lib/Fault Management Blocks/motohawk_fault_def  nam='Lambda_Bank2Bank_Fault'  mode=Enabled  id=[]  x=25  y=50  input_suspected=on  indeterminate=off  increment_xy=on  downsample_count=1  ovr_cals=on  ovr_actions=on  show_actions=on  action1_name=''  action1_cond=(None)  action2_name=''  action2_cond=(None)  action3_name=''  action3_cond=(None)  action4_name=''  action4_cond=(None)
  motohawk_fault_status1 : MotoHawk_lib/Fault Management Blocks/motohawk_fault_status  source=Lookup By Name  nam='Lambda_1_Timeout'  status=Active
  motohawk_fault_status2 : MotoHawk_lib/Fault Management Blocks/motohawk_fault_status  source=Lookup By Name  nam='ECTRangeLow'  status=Active
  motohawk_fault_status3 : MotoHawk_lib/Fault Management Blocks/motohawk_fault_status  source=Lookup By Name  nam='ECTRangeHigh'  status=Active
  motohawk_fault_status9 : MotoHawk_lib/Fault Management Blocks/motohawk_fault_status  source=Lookup By Name  nam='Lambda_2_Timeout'  status=Active
  motohawk_interpolation_2d : MotoHawk_lib/Lookup Tables/motohawk_interpolation_2d  nam='O2Diag_Bank2Bank_DiffAlwd'  table_data=ones(9,9)  show_more=on  data_type=Inherit from 'Table Data'  storage=NonAdaptive  read_level=1  write_level=1  ovr_cals=on  use_help=off  help=''  units=''  use_min_max=off  min_val=-inf  max_val=inf  use_precision=off  precision=''  gain=1  offset=0  exp=1  use_links=off  row_prelookup_block=''  col_prelookup_block=''  output_name=''  use_mototune_group=off  mototune_group=motohawk_vardec_path(gcb)
  wires:
  motohawk_data_read/1 -> Logical Operator33/1
  Logical Operator34/1 -> Logical Operator10/1
  Logical Operator10/1 -> Logical Operator/1
  motohawk_data_read1/1 -> Run State/1
  Run State/1 -> Logical Operator/2
  Sensors/1 -> Bus Selector/1, Bus Selector1/1, Bus Selector2/1, Bus Selector6/1, Bus Selector5/1
  Bus Selector/1 -> Relational Operator/1  "<TimeSinceRun>"
  motohawk_calibration/1 -> Relational Operator/2
  Relational Operator/1 -> Logical Operator/3
  Bus Selector1/1 -> Relational Operator1/1  "<ECT>"
  motohawk_calibration1/1 -> Relational Operator1/2
  Relational Operator1/1 -> Logical Operator/4
  motohawk_fault_status3/1 -> Logical Operator34/1
  motohawk_fault_status2/1 -> Logical Operator34/2
  motohawk_fault_status1/1 -> Logical Operator34/3
  motohawk_fault_status9/1 -> Logical Operator34/4
  Logical Operator33/1 -> Logical Operator34/5
  Logical Operator1/1 -> Logical Operator/5
  Bus Selector2/1 -> Logical Operator1/1  "<DataValidState>"
  Bus Selector2/2 -> Logical Operator1/2  "<DataValidState>"
  DesEquivRatio/1 -> Bus Selector3/1, Bus Selector4/1
  Bus Selector3/1 -> Relational Operator2/1  "<DesEquivRatio>"
  motohawk_calibration2/1 -> Relational Operator2/2
  Relational Operator2/1 -> Logical Operator/6
  Bus Selector4/1 -> Relational Operator3/1  "<DesEquivRatio>"
  motohawk_calibration3/1 -> Relational Operator3/2
  Relational Operator3/1 -> Logical Operator/7
  Bus Selector6/1 -> Sum/1  "<O2_BankA>"
  Bus Selector6/2 -> Sum/2  "<O2_BankB>"
  Sum/1 -> Abs/1
  Abs/1 -> Relational Operator4/1
  motohawk_interpolation_2d/1 -> Relational Operator4/2
  Relational Operator4/1 -> Logical Operator/8
  Logical Operator/1 -> motohawk_fault_def6/1
  Bus Selector5/1 -> motohawk_interpolation_2d/1  "<RPM09Idx>"
  Bus Selector5/2 -> motohawk_interpolation_2d/2  "<MAP09Idx>"
